simulink model "Ornek3_3"  (R2021b)
settings: Solver=VariableStepAuto  StartTime=0.0  StopTime=5  RelTol=1e-3
settings Model: Creator=MONSTER  LastModifiedBy=MONSTER

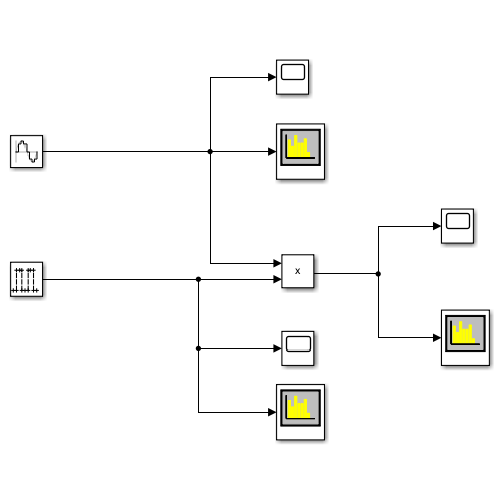
[thumbnail: Simulink's stored preview of the top-level diagram]
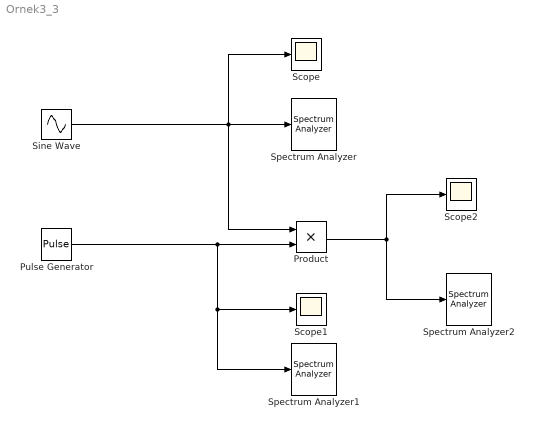
== system Ornek3_3 ==
  Product : Product
  Pulse Generator : DiscretePulseGenerator  Period=5  PulseWidth=4  PhaseDelay=1  SampleTime=0.001
  Scope : Scope
  Scope1 : Scope
  Scope2 : Scope
  Sine Wave : Sin  Frequency=0.3*pi  Phase=0.5*pi  SampleTime=0.001
  Spectrum Analyzer : SpectrumAnalyzer
  Spectrum Analyzer1 : SpectrumAnalyzer
  Spectrum Analyzer2 : SpectrumAnalyzer
  wires:
  Sine Wave/1 -> Product/1, Scope/1, Spectrum Analyzer/1
  Pulse Generator/1 -> Spectrum Analyzer1/1, Scope1/1, Product/2
  Product/1 -> Scope2/1, Spectrum Analyzer2/1
